simulink library "pwrsys"  (R2018a)
settings: Solver=VariableStepAuto  StartTime=0.0  StopTime=10.0  RelTol=1e-3
libraries: $bdroot x1, powerlib_meascontrol x1
Description:
  | NTNU-IEL Power Systems library
settings Model: Creator=ericfa  LastModifiedBy=ericfa

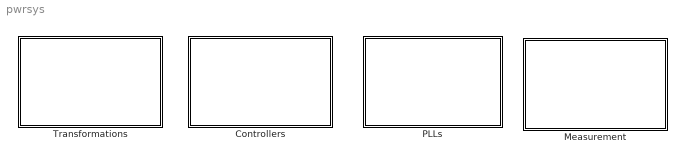
== system pwrsys ==
  Controllers : Subsystem
  Measurement : Subsystem
  PLLs : Subsystem
  Transformations : Subsystem

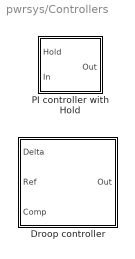
== system pwrsys/Controllers ==
  Droop controller : Subsystem  mask(Droop controller){Refmax=1, Refmin=-1, Kp=1, Kd=0, Tr=0.1, flp=100, DB=0}
      mask prompts: Refmax "Max reference"; Refmin "Min reference"; Kp "Permanent gain"; Kd "Transient gain"; Tr "Reset time [s]"; flp "Low-pass filter cut-off frequency [Hz]"; DB "Dead-band"
      mask help:
      | This block implements a droop controller, i.e. it provides compensation of the input Ref based on the input Delta and Comp.
      |
      | The input Delta is used as input of a PD controller which provides permanent (proportional) and transient (derivative) droop of the input Ref.
      |
      | The input Comp divides the output value of the droop controller and may be used for other types of compensation.
      mask DialogControl DescGroupVar Prompt: Active Power and Frequency Controller
      mask DialogControl DescTextVar Prompt: This block implements a simplified model for power control with droop influence. It can be used either for active power with frequency droop influence or reactive power with voltage droop influence.
      mask DialogControl droop Prompt: Droop control
      mask DialogControl meas Prompt: Delta
  PI controller with Hold : Subsystem  mask(PI controller with anti-windup){Kp=1, Ki=0, Max=1, Min=-1, x0=0}
      mask prompts: Kp "Proportional gain"; Ki "Integral gain"; Max "Maximum output"; Min "Minimum output"; x0 "Initial condition"
      mask help:
      | This block implements a PI controller with anti-windup
      |
      | The input hold freezes the integrator and allows implementing anti-windup in control loops with feed-forward or dynamic limits

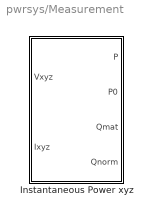
== system pwrsys/Measurement ==
  Instantaneous Power xyz : Subsystem  mask(Instantaneous Power xyz){typeTransf=Amplitude-invariant}
      mask prompts: typeTransf "Type of transformation"
      mask init:
      | switch typeTransf
      |     case 1
      |         a = 1.5;
      |         b = 3;
      |     case 2
      |         a = 1;
      |         b = 1;
      | end
      mask TypeOptions typeTransf: Amplitude-invariant | Power-invariant

== system pwrsys/PLLs ==
  PLL 3-phase abc : Subsystem  mask(3-Phase PLL in the abc frame){fnom=50, fdev=20, zeta=0.707, Kp=100, Ki=50, Kd=10, Tr=100}
      mask prompts: fnom "Rated frequency [Hz]"; fdev "Maximum frequency deviation [Hz]"; zeta "Damping ratio"; Kp "Proportional gain"; Ki "Integral gain"; Kd "Derivative gain"; Tr "Reset time [s]"
      mask help: This block implements a 3-phase PLL in the abc reference frame.
      mask init:
      | wn = fnom/(4*zeta);
      mask DialogControl freqFilter Prompt: Frequency filter
      mask DialogControl ctrl Prompt: Controller

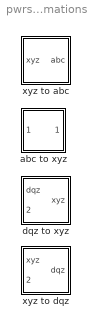
== system pwrsys/Transformations ==
  abc to xyz : Subsystem  mask(Clarke transformation){typeTransf=Amplitude-invariant}
      mask prompts: typeTransf "Type of transformation"
      mask init:
      | switch typeTransf
      |     case 1
      |         a = 1/3;
      |         b = 1/sqrt(3);
      |         c = sqrt(2)/3;
      |     case 2
      |         a = 1/sqrt(6);
      |         b = 1/sqrt(2);
      |         c = 1/sqrt(3);
      | end
      mask TypeOptions typeTransf: Amplitude-invariant | Power-invariant
  dqz to xyz : Subsystem  mask(Inverse Park transformation){}
  xyz to abc : Subsystem  mask(Inverse Clarke transformation){typeTransf=Amplitude-invariant}
      mask prompts: typeTransf "Type of transformation"
      mask init:
      | switch typeTransf
      |     case 1
      |         a = 1;
      |         b = sqrt(3)/2;
      |         c = 1/2;
      |         d = 1/sqrt(2);
      |     case 2
      |         a = sqrt(2/3);
      |         b = 1/sqrt(2);
      |         c = 1/sqrt(6);
      |         d = 1/sqrt(3);
      | end
      mask TypeOptions typeTransf: Amplitude-invariant | Power-invariant
  xyz to dqz : Subsystem  mask(Inverse Park transformation){}

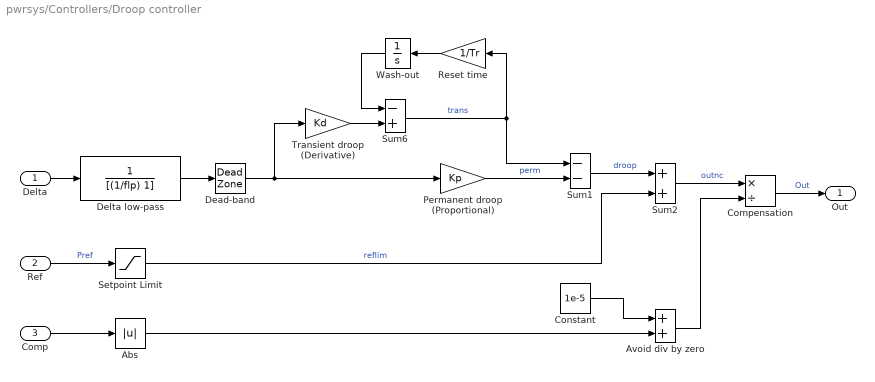
== system pwrsys/Controllers/Droop controller ==
  Delta : Inport
  Ref : Inport  Port=2
  Comp : Inport  Port=3
  Abs : Abs  ZeroCross=off
  Avoid div by zero : Sum
  Compensation : Product  Inputs=*/
  Constant : Constant  Value=1e-5
  Dead-band : DeadZone  LowerValue=-DB  UpperValue=DB  SaturateOnIntegerOverflow=on
  Delta low-pass : TransferFcn  Denominator=[(1/flp) 1]
  Permanent droop (Proportional) : Gain  Gain=Kp
  Reset time : Gain  Gain=1/Tr
  Setpoint Limit : Saturate  UpperLimit=Refmax  LowerLimit=Refmin  ZeroCross=off
  Sum1 : Sum  Inputs=--
  Sum2 : Sum
  Sum6 : Sum  Inputs=-+
  Transient droop (Derivative) : Gain  Gain=Kd
  Wash-out : Integrator  LimitOutput=on  UpperSaturationLimit=1  LowerSaturationLimit=-1  ZeroCross=off
  Out : Outport
  wires:
  Permanent droop (Proportional)/1 -> Sum1/2  "perm"
  Wash-out/1 -> Sum6/1
  Transient droop (Derivative)/1 -> Sum6/2
  Sum1/1 -> Sum2/1  "droop"
  Sum6/1 -> Sum1/1, Reset time/1  "trans"
  Reset time/1 -> Wash-out/1
  Delta/1 -> Delta low-pass/1
  Ref/1 -> Setpoint Limit/1  "Pref"
  Sum2/1 -> Compensation/1  "outnc"
  Delta low-pass/1 -> Dead-band/1
  Dead-band/1 -> Permanent droop (Proportional)/1, Transient droop (Derivative)/1
  Comp/1 -> Abs/1
  Setpoint Limit/1 -> Sum2/2  "reflim"
  Constant/1 -> Avoid div by zero/1
  Avoid div by zero/1 -> Compensation/2
  Compensation/1 -> Out/1  "Out"
  Abs/1 -> Avoid div by zero/2

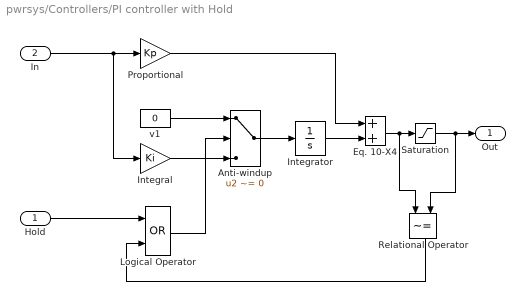
== system pwrsys/Controllers/PI controller with Hold ==
  Hold : Inport
  In : Inport  Port=2
  Anti-windup : Switch  Criteria=u2 ~= 0
  Eq. 10-X4 : Sum  SaturateOnIntegerOverflow=on  InputSameDT=on  OutDataTypeStr=Inherit: Same as first input
  Integral : Gain  Gain=Ki
  Integrator : Integrator  InitialCondition=x0  UpperSaturationLimit=0  LowerSaturationLimit=0
  Logical Operator : Logic  Operator=OR  AllPortsSameDT=off  OutDataTypeStr=boolean
  Proportional : Gain  Gain=Kp
  Relational Operator : RelationalOperator  Operator=~=  OutDataTypeStr=boolean  RndMeth=Simplest
  Saturation : Saturate  UpperLimit=Max  LowerLimit=Min
  v1 : Constant  Value=0
  Out : Outport
  wires:
  Integrator/1 -> Eq. 10-X4/2
  Integral/1 -> Anti-windup/3
  Anti-windup/1 -> Integrator/1
  Hold/1 -> Logical Operator/1
  In/1 -> Integral/1, Proportional/1
  Eq. 10-X4/1 -> Saturation/1, Relational Operator/1
  v1/1 -> Anti-windup/1
  Saturation/1 -> Relational Operator/2, Out/1
  Relational Operator/1 -> Logical Operator/2
  Logical Operator/1 -> Anti-windup/2
  Proportional/1 -> Eq. 10-X4/1

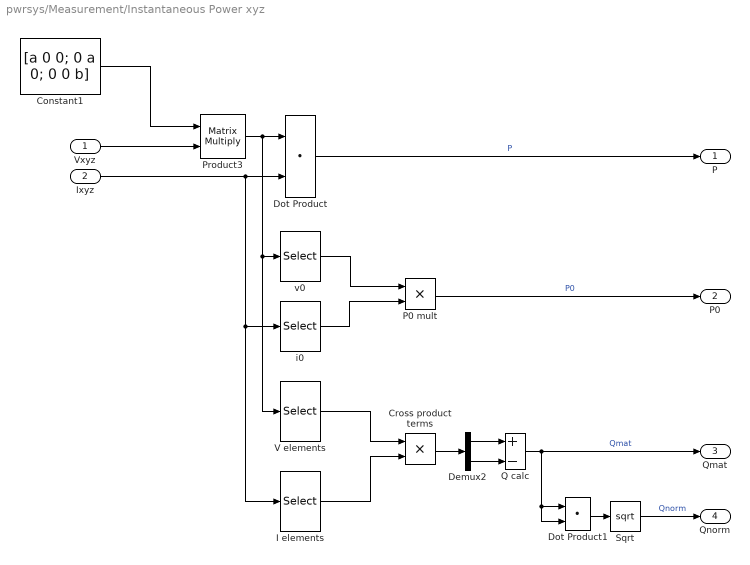
== system pwrsys/Measurement/Instantaneous Power xyz ==
  Vxyz : Inport
  Ixyz : Inport  Port=2
  Constant1 : Constant  Value=[a 0 0; 0 a 0; 0 0 b]
  Cross product terms : Product  RndMeth=Zero
  Demux2 : Demux  Outputs=2
  Dot Product : DotProduct  InputSameDT=on  OutDataTypeStr=Inherit: Inherit via internal rule
  Dot Product1 : DotProduct  InputSameDT=on  OutDataTypeStr=Inherit: Inherit via internal rule
  I elements : Selector  InputPortWidth=3  IndexOptions=Index vector (dialog)  Indices=[3 1 2 2 3 1]  OutputSizes=1
  P0 mult : Product  RndMeth=Zero
  Product3 : Product  Multiplication=Matrix(*)
  Q calc : Sum  Inputs=+-
  Sqrt : Sqrt  SaturateOnIntegerOverflow=on
  V elements : Selector  InputPortWidth=3  IndexOptions=Index vector (dialog)  Indices=[2 3 1 3 1 2]  OutputSizes=1
  i0 : Selector  InputPortWidth=3  IndexOptions=Index vector (dialog)  Indices=[3]  OutputSizes=1
  v0 : Selector  InputPortWidth=3  IndexOptions=Index vector (dialog)  Indices=[3]  OutputSizes=1
  P : Outport
  P0 : Outport  Port=2
  Qmat : Outport  Port=3
  Qnorm : Outport  Port=4
  wires:
  Dot Product/1 -> P/1  "P"
  Q calc/1 -> Qmat/1, Dot Product1/2, Dot Product1/1  "Qmat"
  Constant1/1 -> Product3/1
  Product3/1 -> V elements/1, v0/1, Dot Product/1
  Demux2/1 -> Q calc/1
  I elements/1 -> Cross product terms/2
  Vxyz/1 -> Product3/2
  Demux2/2 -> Q calc/2
  Ixyz/1 -> I elements/1, i0/1, Dot Product/2
  V elements/1 -> Cross product terms/1
  Cross product terms/1 -> Demux2/1
  v0/1 -> P0 mult/1
  i0/1 -> P0 mult/2
  P0 mult/1 -> P0/1  "P0"
  Dot Product1/1 -> Sqrt/1
  Sqrt/1 -> Qnorm/1  "Qnorm"

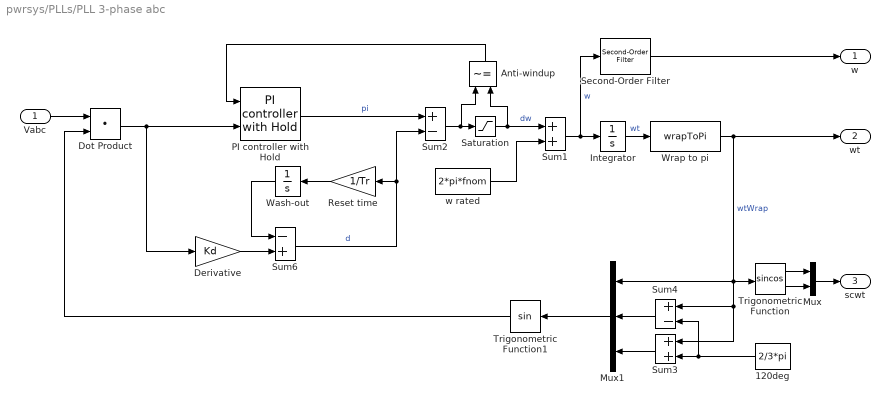
== system pwrsys/PLLs/PLL 3-phase abc ==
  Vabc : Inport
  120deg : Constant  Value=2/3*pi
  Anti-windup : RelationalOperator  Operator=~=  OutDataTypeStr=boolean  RndMeth=Simplest
  Derivative : Gain  Gain=Kd
  Dot Product : DotProduct  InputSameDT=on  OutDataTypeStr=Inherit: Inherit via internal rule
  Integrator : Integrator  UpperSaturationLimit=1  LowerSaturationLimit=-1  ZeroCross=off
  Mux : Mux  Inputs=2
  Mux1 : Mux  Inputs=3
  PI controller with Hold : $bdroot/Controllers/PI controller  with Hold  Kp=Kp  Ki=Ki  Max=2*pi*fdev  Min=-2*pi*fdev  x0=0
  Reset time : Gain  Gain=1/Tr
  Saturation : Saturate  UpperLimit=2*pi*fdev  LowerLimit=-2*pi*fdev
  Second-Order Filter : powerlib_meascontrol/Filters/Second-Order Filter  FilterType=Lowpass  Fo=wn  Zeta=zeta  Ts=0  Initialize=on  Vac_Init="[0,  0,  60]"  Vdc_Init=2*pi*fnom  PlotResponse=off  FreqRange=[0, 500, 1]
      settings: SourceProductName=Simscape Power Systems  SourceProductBaseCode=PS
  Sum1 : Sum
  Sum2 : Sum  Inputs=+-
  Sum3 : Sum
  Sum4 : Sum  Inputs=+-
  Sum6 : Sum  Inputs=-+
  Trigonometric Function : Trigonometry  Operator=sincos  ApproximationMethod=CORDIC
  Trigonometric Function1 : Trigonometry  ApproximationMethod=CORDIC
  Wash-out : Integrator  LimitOutput=on  UpperSaturationLimit=2*pi*fdev  LowerSaturationLimit=-2*pi*fdev  ZeroCross=off
  Wrap to pi : MATLABFcn  MATLABFcn=wrapToPi
  w rated : Constant  Value=2*pi*fnom
  w : Outport
  wt : Outport  Port=2
  scwt : Outport  Port=3
  wires:
  Reset time/1 -> Wash-out/1
  Wash-out/1 -> Sum6/1
  Sum6/1 -> Sum2/2, Reset time/1  "d"
  Derivative/1 -> Sum6/2
  Saturation/1 -> Sum1/1, Anti-windup/2  "dw"
  w rated/1 -> Sum1/2
  Sum1/1 -> Second-Order Filter/1, Integrator/1  "w"
  Integrator/1 -> Wrap to pi/1  "wt"
  Vabc/1 -> Dot Product/1
  PI controller with Hold/1 -> Sum2/1  "pi"
  Sum2/1 -> Anti-windup/1, Saturation/1
  Anti-windup/1 -> PI controller with Hold/1
  Wrap to pi/1 -> Mux1/1, Trigonometric Function/1, Sum4/1, Sum3/1, wt/1  "wtWrap"
  Trigonometric Function/1 -> Mux/1
  Trigonometric Function/2 -> Mux/2
  Mux/1 -> scwt/1
  120deg/1 -> Sum4/2, Sum3/2
  Sum4/1 -> Mux1/2
  Sum3/1 -> Mux1/3
  Mux1/1 -> Trigonometric Function1/1
  Trigonometric Function1/1 -> Dot Product/2
  Second-Order Filter/1 -> w/1
  Dot Product/1 -> Derivative/1, PI controller with Hold/2

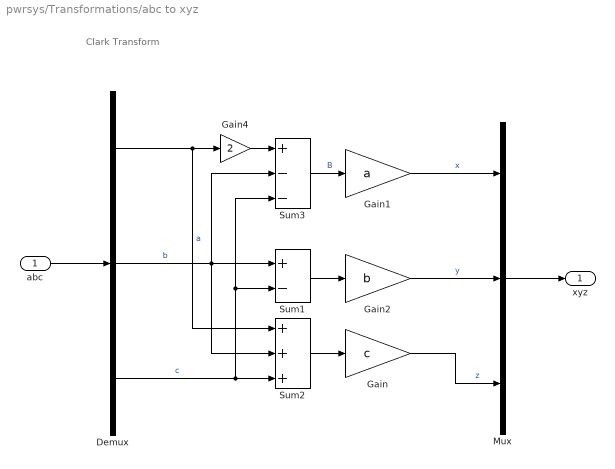
== system pwrsys/Transformations/abc to xyz ==
  note: Clark Transform
  abc : Inport
  Demux : Demux  Outputs=3
  Gain : Gain  Gain=c
  Gain1 : Gain  Gain=a
  Gain2 : Gain  Gain=b
  Gain4 : Gain  Gain=2
  Mux : Mux  Inputs=3
  Sum1 : Sum  Inputs=+-
  Sum2 : Sum  Inputs=+++
  Sum3 : Sum  Inputs=+--
  xyz : Outport
  wires:
  abc/1 -> Demux/1
  Demux/1 -> Sum2/1, Gain4/1  "a"
  Gain/1 -> Mux/3  "z"
  Gain2/1 -> Mux/2  "y"
  Gain1/1 -> Mux/1  "x"
  Mux/1 -> xyz/1
  Gain4/1 -> Sum3/1
  Demux/2 -> Sum2/2, Sum1/1, Sum3/2  "b"
  Demux/3 -> Sum2/3, Sum1/2, Sum3/3  "c"
  Sum3/1 -> Gain1/1  "B"
  Sum1/1 -> Gain2/1
  Sum2/1 -> Gain/1

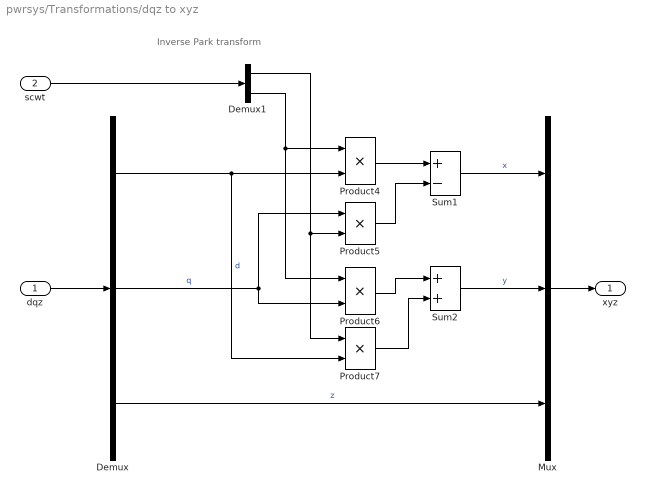
== system pwrsys/Transformations/dqz to xyz ==
  note: Inverse Park transform
  dqz : Inport
  scwt : Inport  Port=2
  Demux : Demux  Outputs=3
  Demux1 : Demux  Outputs=2
  Mux : Mux  Inputs=3
  Product{4..7} (4 alike) : Product
  Sum1 : Sum  Inputs=+-
  Sum2 : Sum
  xyz : Outport
  wires:
  dqz/1 -> Demux/1
  Demux/1 -> Product7/2, Product4/2  "d"
  Demux1/2 -> Product4/1, Product6/1
  Product5/1 -> Sum1/2
  Product4/1 -> Sum1/1
  Demux1/1 -> Product7/1, Product5/2
  Demux/2 -> Product6/2, Product5/1  "q"
  scwt/1 -> Demux1/1
  Product6/1 -> Sum2/1
  Product7/1 -> Sum2/2
  Mux/1 -> xyz/1
  Demux/3 -> Mux/3  "z"
  Sum2/1 -> Mux/2  "y"
  Sum1/1 -> Mux/1  "x"

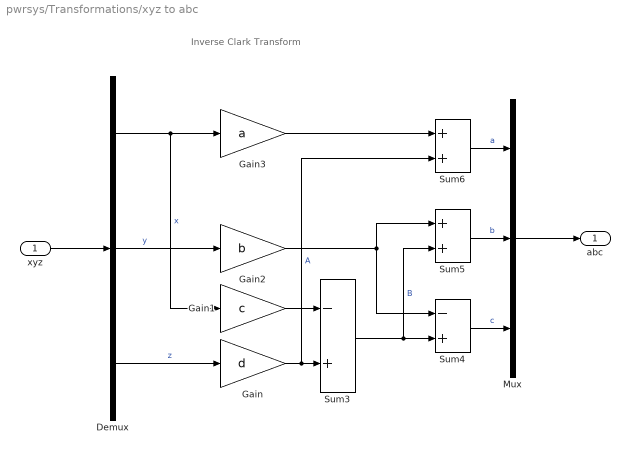
== system pwrsys/Transformations/xyz to abc ==
  note: Inverse Clark Transform
  xyz : Inport
  Demux : Demux  Outputs=3
  Gain : Gain  Gain=d
  Gain1 : Gain  Gain=c
  Gain2 : Gain  Gain=b
  Gain3 : Gain  Gain=a
  Mux : Mux  Inputs=3
  Sum3 : Sum  Inputs=-+
  Sum4 : Sum  Inputs=-+
  Sum5 : Sum
  Sum6 : Sum
  abc : Outport
  wires:
  xyz/1 -> Demux/1
  Demux/2 -> Gain2/1  "y"
  Demux/1 -> Gain3/1, Gain1/1  "x"
  Demux/3 -> Gain/1  "z"
  Gain1/1 -> Sum3/1
  Gain/1 -> Sum6/2, Sum3/2  "A"
  Gain2/1 -> Sum5/1, Sum4/1
  Sum3/1 -> Sum5/2, Sum4/2  "B"
  Sum4/1 -> Mux/3  "c"
  Sum5/1 -> Mux/2  "b"
  Sum6/1 -> Mux/1  "a"
  Gain3/1 -> Sum6/1
  Mux/1 -> abc/1

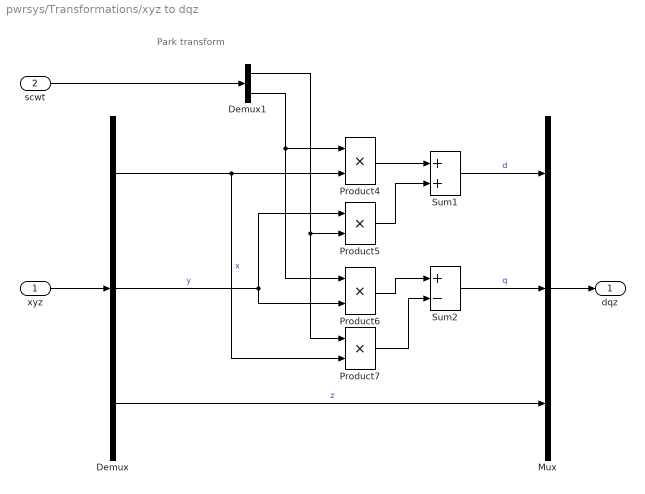
== system pwrsys/Transformations/xyz to dqz ==
  note: Park transform
  xyz : Inport
  scwt : Inport  Port=2
  Demux : Demux  Outputs=3
  Demux1 : Demux  Outputs=2
  Mux : Mux  Inputs=3
  Product{4..7} (4 alike) : Product
  Sum1 : Sum
  Sum2 : Sum  Inputs=+-
  dqz : Outport
  wires:
  Sum1/1 -> Mux/1  "d"
  Sum2/1 -> Mux/2  "q"
  Demux/3 -> Mux/3  "z"
  Mux/1 -> dqz/1
  Product7/1 -> Sum2/2
  Product6/1 -> Sum2/1
  scwt/1 -> Demux1/1
  Demux/2 -> Product5/1, Product6/2  "y"
  Demux1/1 -> Product5/2, Product7/1
  Product4/1 -> Sum1/1
  Product5/1 -> Sum1/2
  Demux1/2 -> Product6/1, Product4/1
  Demux/1 -> Product4/2, Product7/2  "x"
  xyz/1 -> Demux/1
